simulink model "uncontrolled_response"  (R2024a)
settings: Solver=VariableStepAuto  StartTime=0.0  StopTime=2  FixedStep=1e-6  MaxStep=1e-3  RelTol=1e-3
values from neighbouring files (symbols this model uses):
  B = 0.068    [parameters.m]
  h = 0.009    [parameters.m]
  J = 0.51    [parameters.m]
  r = 4    [parameters.m]
libraries: DEMDlib x3
settings Model: Creator=roberto  LastModifiedBy=roberto
settings DebuggingCC: ReadBeforeWriteMsg=DisableAll  WriteAfterWriteMsg=DisableAll  WriteAfterReadMsg=DisableAll  MultiTaskDSMMsg=none
settings ModelReferenceCC: UpdateModelReferenceTargets=IfOutOfDate
settings SFSimCC: SFSimEcho=off

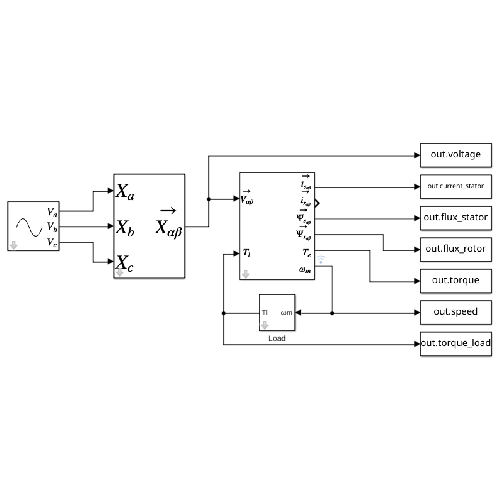
[thumbnail: Simulink's stored preview of the top-level diagram]
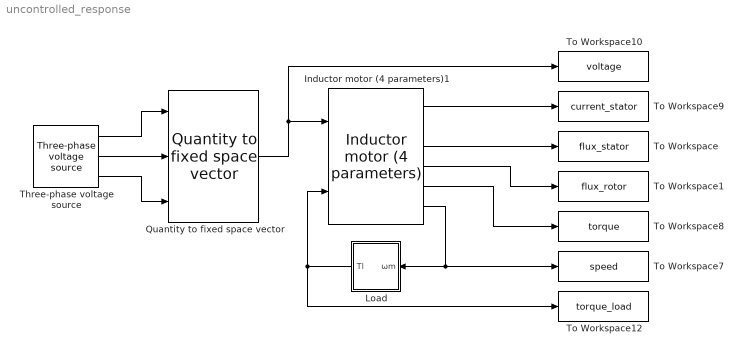
== system uncontrolled_response ==
  Inductor motor (4 parameters)1 : DEMDlib/Inductor motor (4 parameters)  Rs=Rs  Lks=Lks  Rr=Rkr  Lm=Lkm  np=np  J=J  B=B
      settings: SourceProductName=DEMD
  Load : Subsystem  mask(Quadratic load){r=r, k=h}
      mask DialogControl Control2 Prompt: Ratio (ωl/ωm)
      mask DialogControl Control2_copy Prompt: Load proportional coefficient (Nm s^2 / rad^2)
  Quantity to fixed space vector : DEMDlib/Quantity to fixed space vector
      settings: SourceProductName=DEMD
  Three-phase voltage source : DEMDlib/Power suply/Three-phase voltage source  Vac=Vac  fac=fac
      settings: SourceProductName=DEMD
  To Workspace : ToWorkspace  VariableName=flux_stator  SaveFormat=Timeseries  SampleTime=-1
  To Workspace1 : ToWorkspace  VariableName=flux_rotor  SaveFormat=Timeseries  SampleTime=-1
  To Workspace10 : ToWorkspace  VariableName=voltage  SaveFormat=Timeseries  SampleTime=-1
  To Workspace12 : ToWorkspace  VariableName=torque_load  SaveFormat=Timeseries  SampleTime=-1
  To Workspace7 : ToWorkspace  VariableName=speed  SaveFormat=Timeseries  SampleTime=-1
  To Workspace8 : ToWorkspace  VariableName=torque  SaveFormat=Timeseries  SampleTime=-1
  To Workspace9 : ToWorkspace  VariableName=current_stator  SaveFormat=Timeseries  SampleTime=-1
  wires:
  Three-phase voltage source/3 -> Quantity to fixed space vector/3
  Three-phase voltage source/2 -> Quantity to fixed space vector/2
  Three-phase voltage source/1 -> Quantity to fixed space vector/1
  Inductor motor (4 parameters)1/1 -> To Workspace9/1
  Inductor motor (4 parameters)1/3 -> To Workspace/1
  Inductor motor (4 parameters)1/5 -> To Workspace8/1
  Quantity to fixed space vector/1 -> Inductor motor (4 parameters)1/1, To Workspace10/1
  Inductor motor (4 parameters)1/4 -> To Workspace1/1
  Inductor motor (4 parameters)1/6 -> To Workspace7/1, Load/1(ωm)
  Load/1(Tl) -> Inductor motor (4 parameters)1/2, To Workspace12/1

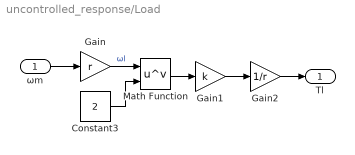
== system uncontrolled_response/Load ==
  ωm : Inport
  Constant3 : Constant  Value=2
  Gain : Gain  Gain=r
  Gain1 : Gain  Gain=k
  Gain2 : Gain  Gain=1/r
  Math Function : Math  Operator=pow
  Tl : Outport
  wires:
  Gain/1 -> Math Function/1  "ωl"
  Constant3/1 -> Math Function/2
  Math Function/1 -> Gain1/1
  Gain1/1 -> Gain2/1
  Gain2/1 -> Tl/1
  ωm/1 -> Gain/1
